simulink model "rSOCDerate"  (R2024b)
settings: configuration reference "STM32H7_Config" (kept outside this file)
settings Model: DataDictionary=Master_Dictionary.sldd  EnableAccessToBaseWorkspace=off  Creator=torni  LastModifiedBy=William
settings ConfigSetRef: SourceName=STM32H7_Config

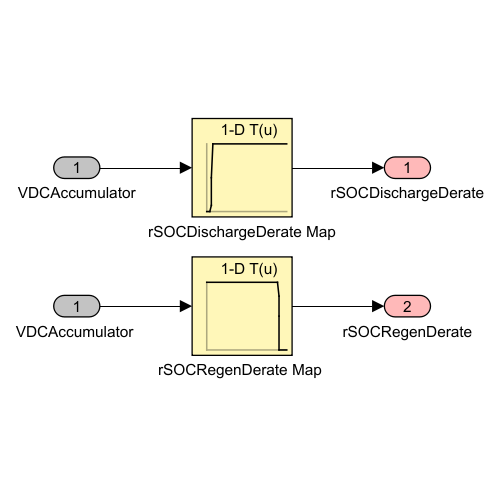
[thumbnail: Simulink's stored preview of the top-level diagram]
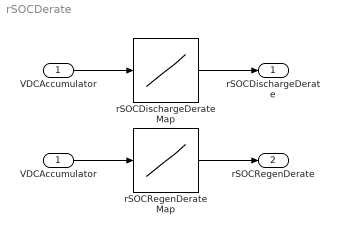
== system rSOCDerate ==
  VDCAccumulator : Inport  OutDataTypeStr=double
  "VDCAccumulator " : InportShadow  OutDataTypeStr=double
  rSOCDischargeDerate Map : Lookup_n-D  NumberOfTableDimensions=1  BreakpointsForDimension1=[380,390,392,395,396,600]  Table=[0,0,0.1,0.5,1,1]  InternalRulePriority=Speed  RndMeth=Simplest
  "rSOCRegenDerate Map " : Lookup_n-D  NumberOfTableDimensions=1  BreakpointsForDimension1=[0,535,540,542,544,600]  Table=[1,1,0.8,0.5,0,0]  InternalRulePriority=Speed  RndMeth=Simplest
  rSOCDischargeDerate : Outport  OutDataTypeStr=double  VectorParamsAs1DForOutWhenUnconnected=off
  rSOCRegenDerate : Outport  Port=2  OutDataTypeStr=double  VectorParamsAs1DForOutWhenUnconnected=off
  wires:
  VDCAccumulator/1 -> rSOCDischargeDerate Map/1
  rSOCDischargeDerate Map/1 -> rSOCDischargeDerate/1
  "rSOCRegenDerate Map "/1 -> rSOCRegenDerate/1
  "VDCAccumulator "/1 -> "rSOCRegenDerate Map "/1
